simulink model "transfer_func"  (R2016a)
settings: Solver=FixedStepAuto  StartTime=0.0  StopTime=2  FixedStep=0.001  RelTol=1e-3
settings Model: Creator=marki  LastModifiedBy=marki

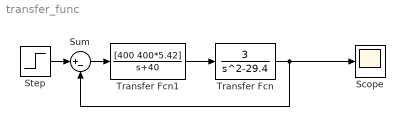
== system transfer_func ==
  Scope : Scope
  Step : Step  After=0.05  SampleTime=0
  Sum : Sum  Inputs=|+-
  Transfer Fcn : TransferFcn  Numerator=[3]  Denominator=[1 0 -29.4]
  Transfer Fcn1 : TransferFcn  Numerator=[400 400*5.42]  Denominator=[ 1 40]
  wires:
  Step/1 -> Sum/1
  Transfer Fcn/1 -> Scope/1, Sum/2
  Transfer Fcn1/1 -> Transfer Fcn/1
  Sum/1 -> Transfer Fcn1/1
